simulink model "Model"  (R2015a)
settings: Solver=ode45  StartTime=0.0  StopTime=10.0  RelTol=1e-3
settings Model: CovSFcnEnable=off  Creator=qiji  LastModifiedBy=qiji
settings DebuggingCC: UnderspecifiedInitializationDetection=Classic  MergeDetectMultiDrivingBlocksExec=none  SolverPrmCheckMsg=warning

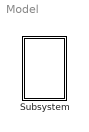
== system Model ==
  Subsystem : Subsystem

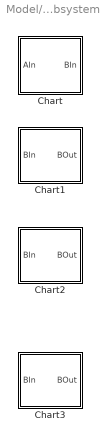
== system Model/Subsystem ==
  Chart : Stateflow chart  TreatAsAtomicUnit=on
  Chart1 : Stateflow chart  TreatAsAtomicUnit=on
  Chart2 : Stateflow chart  TreatAsAtomicUnit=on
  Chart3 : Stateflow chart  TreatAsAtomicUnit=on

== stateflow chart Model/Subsystem/Chart ==
  state A
    en:
    AOut = 0;
  state B
    en:
    AOut = 1;
  A -> B : [AIn == 1]
  (default) -> A
  B -> A : [AIn==1]
  data: AIn input double; BIn output double
  data AIn settings: description=in

== stateflow chart Model/Subsystem/Chart1 ==
  state A
    du:
    BOut = BIn
  (default) -> A
  data: BOut output double; BIn input double
  data BOut settings: description=out

== stateflow chart Model/Subsystem/Chart2 ==
  state A
    du:
    BOut = BIn
  (default) -> A
  data: BOut output double; BIn input double
  data BOut settings: description=out

== stateflow chart Model/Subsystem/Chart3 ==
  state A
    du:
    BOut = BIn
  (default) -> A
  data: BOut output double; BIn input double
  data BOut settings: description=out
